simulink model "model_simscape"  (R2021a)
settings: Solver=VariableStepAuto  StartTime=0.0  StopTime=10  FixedStep=Ts  RelTol=1e-3
values from neighbouring files (symbols this model uses):
  acc_C = -1/g    (= -0.101936799185)    [params.m]
  acc_enable = 1    [params.m]
  acc_noise_var = 1e-10    [params.m]
  B_hs = 1e5    (= 100000)    [params.m]
  b_small_bot = 1400    [params.m]
  b_small_up = 1417.14082244839    (= 1417.14082245)    [params.m]
  beta = 0    [params.m]
  flow_C = flow_enable/flow_C_ratio/conv_SI    (= 59999.988)    [params.m]
  flow_C_ratio = dm_max/U_f_max    (= 1)    [params.m]
  flow_noise_var = 1e-10    [params.m]
  g = 9.81    [params.m]
  K_hs = 1e5    (= 100000)    [params.m]
  L = NaN(N,nk)    [hammerstein_wiener_model_estimation.m]    (also in params.m = 0.2)
  M = 6.7798462575453    (= 6.77984625755)    [params.m]
  M_L = member.("Settings.Load"){1,1}{1,1}    [identification_faultcode.m]    (also in params.m = 6.25)
  P_0 = 101325    [params.m]
  P_s = 6e5    (= 600000)    [params.m]
  prox_bot_band = 4e-4    (= 0.0004)    [params.m]
  prox_up_band = 0.1925    [params.m]
  SmallDamper_bottom = member.SmallDamper_bottom{1,1}.Variables    [identification_faultcode.m]    (also in params.m = 6)
  SmallDamper_upper = member.SmallDamper_upper{1,1}.Variables    [identification_faultcode.m]    (also in params.m = 4)
  T = cell2mat(T)    [data_driven_models_perfomance.m]    (also in params.m = 281.7)
  Ts = 1e-3    (= 0.001)    [data_driven_models_perfomance.m]    (also in hammerstein_wiener_model_estimation.m; params.m)
  valve1 = member.ThrottleValve2{1,1}.Variables    [identification_faultcode.m]    (also in params.m = 4)
  valve2 = member.ThrottleValve1{1,1}.Variables    [identification_faultcode.m]    (also in params.m = 6)
  x0 = 0    [params.m]
libraries: fl_lib x20, nesl_utility x14, SimscapeFluids_lib x6
(part 2 of 2)

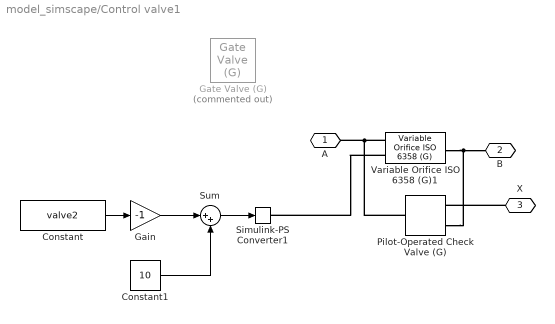
== system model_simscape/Control valve1 ==
  Constant : Constant  Value=valve2
  Constant1 : Constant  Value=10
  Gain : Gain  Gain=-1
  Gate Valve (G) : SimscapeFluids_lib/Gas/Valves & Orifices/Flow Control Valves/Gate Valve (G)  Commented=on  diam_orifice=d_G18 m  x0=0  iso_cond_spec=fluids.gas.enum.flow_control_valve_spec.Cv  C_max=1.6 l/s/bar  B_crit=0.3  m=0.5  Cv_max=0.53  Kv_max=0.3  area_leak=1e-12 m^2  area=cs_G18 m^2  smoothing_factor=0  B_lam=B_lam  T0=T K  rho0=rho kg/m^3
      settings: SourceProductBaseCode=SH  InternalSimscapePortConfiguration="{\"Bottom\":[],\"Left\":[{\"id\":\"A\",\"label\":\"A\",\"type\":\"foundation.gas.gas\"},{\"id\":\"L\",\"label\":\"L\",\"type\":\"input\"}],\"Right\":[{\"id\":\"B\",\"label\":\"B\",\"type\":\"foundation.gas.gas\"}],\"Top\":[]}"
  Pilot-Operated Check Valve (G) : SimscapeFluids_lib/Gas/Valves & Orifices/Directional Control Valves/Pilot-Operated Check Valve (G)  pressure_spec=fluids.gas.enum.pilot_pressure_control_spec.dp  p_crack_differential=6 bar  press_max_differential=7 bar  pilot_ratio=1  iso_cond_spec=fluids.gas.enum.iso_cond_spec.Kv  C_max=1.6 l/s/bar  C_min=1e-5 l/s/bar  B_crit=0.3  m=0.5  Cv_max=0.38  Cv_min=1e-6  Kv_max=0.3287  Kv_min=1e-6  area_max=1e-4 m^2  area_leak=1e-12 m^2  area=0.01 m^2  smoothing_factor=0  B_lam=0.999  T0=293.15 K  rho0=1.185 kg/m^3
      settings: SourceProductBaseCode=SH  InternalSimscapePortConfiguration="{\"Bottom\":[],\"Left\":[{\"id\":\"A\",\"label\":\"A\",\"type\":\"foundation.gas.gas\"},{\"id\":\"X\",\"label\":\"X\",\"type\":\"foundation.gas.gas\"}],\"Right\":[{\"id\":\"B\",\"label\":\"B\",\"type\":\"foundation.gas.gas\"}],\"Top\":[]}"
  Simulink-PS Converter1 : nesl_utility/Simulink-PS Converter  PhysicalDomain=network_engine_domain  SubClassName=ps_input  LeftPortType=input  RightPortType=output  PseudoPeriodic=off  Frequencies=[]  NoiseDistribution=none  NoiseParameters=[]  Unit=1  AffineConversion=off  FilteringAndDerivatives=provide  SimscapeFilterOrder=1  InputFilterTimeConstant=0.001  UdotUserProvided=0
      settings: SourceProductBaseCode=PW,SS
  Sum : Sum  Inputs=|++
  Variable Orifice ISO 6358 (G)1 : SimscapeFluids_lib/Gas/Valves & Orifices/Variable Orifice ISO 6358 (G)  iso_cond_spec=fluids.gas.enum.iso_cond_spec.Kv  iso_opening_spec_C=fluids.gas.enum.iso_opening_spec.linear  C_max=1.6 l/s/bar  C_min=1e-5 l/s/bar  B_crit=0.3  opening_C_TLU=0 : 0.2 : 1  C_TLU=[1e-05, .32, .64, .96, 1.28, 1.6] l/s/bar  B_crit_TLU=0.3 * ones(1, 6)  m=0.5  iso_opening_spec_Cv=fluids.gas.enum.iso_opening_spec.tabulated  Cv_max=0.4  Cv_min=1e-6  opening_Cv_TLU=0 : 0.2 : 1  Cv_TLU=[1e-06, .08, .16, .24, .32, .4]  iso_opening_spec_Kv=fluids.gas.enum.iso_opening_spec.tabulated  Kv_max=0.1038  Kv_min=Kv_min_cntr  opening_Kv_TLU=lookup_n  Kv_TLU=lookup_qn_Kv  iso_opening_spec_area=fluids.gas.enum.iso_opening_spec.linear  restriction_area_max=1e-5 m^2  restriction_area_min=1e-10 m^2  opening_area_TLU=0 : 0.2 : 1  restriction_area_TLU=[1e-10, 2e-06, 4e-06, 6e-06, 8e-06, 1e-05] m^2  area=cs_G18 m^2  B_lam=0.999  T0=T K  rho0=rho kg/m^3  smoothing_factor=0
      settings: SourceProductBaseCode=SH  InternalSimscapePortConfiguration="{\"Bottom\":[],\"Left\":[{\"id\":\"A\",\"label\":\"A\",\"type\":\"foundation.gas.gas\"},{\"id\":\"L\",\"label\":\"L\",\"type\":\"input\"}],\"Right\":[{\"id\":\"B\",\"label\":\"B\",\"type\":\"foundation.gas.gas\"}],\"Top\":[]}"
  A : PMIOPort  Side=Left
  B : PMIOPort  Port=2  Side=Right
  X : PMIOPort  Port=3  Side=Left
  wires:
  Sum/1 -> Simulink-PS Converter1/1
  Gain/1 -> Sum/1
  Constant/1 -> Gain/1
  Constant1/1 -> Sum/2
  connections:
  Variable Orifice ISO 6358 (G)1/LConn1 -- Pilot-Operated Check Valve (G)/RConn1 -- A/RConn1
  Variable Orifice ISO 6358 (G)1/RConn1 -- Pilot-Operated Check Valve (G)/LConn1 -- B/RConn1
  Variable Orifice ISO 6358 (G)1/LConn2 -- Simulink-PS Converter1/RConn1
  X/RConn1 -- Pilot-Operated Check Valve (G)/LConn2

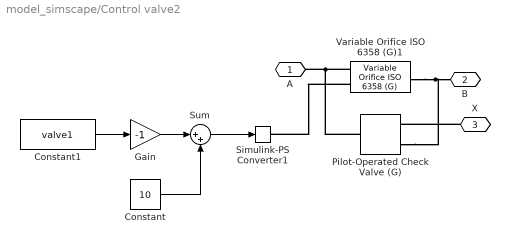
== system model_simscape/Control valve2 ==
  Constant : Constant  Value=10
  Constant1 : Constant  Value=valve1
  Gain : Gain  Gain=-1
  Pilot-Operated Check Valve (G) : SimscapeFluids_lib/Gas/Valves & Orifices/Directional Control Valves/Pilot-Operated Check Valve (G)  pressure_spec=fluids.gas.enum.pilot_pressure_control_spec.dp  p_crack_differential=6 bar  press_max_differential=7 bar  pilot_ratio=1  iso_cond_spec=fluids.gas.enum.iso_cond_spec.Kv  C_max=1.6 l/s/bar  C_min=1e-5 l/s/bar  B_crit=0.3  m=0.5  Cv_max=0.4  Cv_min=1e-6  Kv_max=0.3287  Kv_min=1e-6  area_max=1e-4 m^2  area_leak=1e-12 m^2  area=0.01 m^2  smoothing_factor=0  B_lam=0.999  T0=293.15 K  rho0=1.185 kg/m^3
      settings: SourceProductBaseCode=SH  InternalSimscapePortConfiguration="{\"Bottom\":[],\"Left\":[{\"id\":\"A\",\"label\":\"A\",\"type\":\"foundation.gas.gas\"},{\"id\":\"X\",\"label\":\"X\",\"type\":\"foundation.gas.gas\"}],\"Right\":[{\"id\":\"B\",\"label\":\"B\",\"type\":\"foundation.gas.gas\"}],\"Top\":[]}"
  Simulink-PS Converter1 : nesl_utility/Simulink-PS Converter  PhysicalDomain=network_engine_domain  SubClassName=ps_input  LeftPortType=input  RightPortType=output  PseudoPeriodic=off  Frequencies=[]  NoiseDistribution=none  NoiseParameters=[]  Unit=1  AffineConversion=off  FilteringAndDerivatives=provide  SimscapeFilterOrder=1  InputFilterTimeConstant=0.001  UdotUserProvided=0
      settings: SourceProductBaseCode=PW,SS
  Sum : Sum  Inputs=|++
  Variable Orifice ISO 6358 (G)1 : SimscapeFluids_lib/Gas/Valves & Orifices/Variable Orifice ISO 6358 (G)  iso_cond_spec=fluids.gas.enum.iso_cond_spec.Kv  iso_opening_spec_C=fluids.gas.enum.iso_opening_spec.linear  C_max=1.6 l/s/bar  C_min=1e-5 l/s/bar  B_crit=0.3  opening_C_TLU=0 : 0.2 : 1  C_TLU=[1e-05, .32, .64, .96, 1.28, 1.6] l/s/bar  B_crit_TLU=0.3 * ones(1, 6)  m=0.5  iso_opening_spec_Cv=fluids.gas.enum.iso_opening_spec.tabulated  Cv_max=0.4  Cv_min=1e-6  opening_Cv_TLU=0 : 0.2 : 1  Cv_TLU=[1e-06, .08, .16, .24, .32, .4]  iso_opening_spec_Kv=fluids.gas.enum.iso_opening_spec.tabulated  Kv_max=0.1038  Kv_min=Kv_min_cntr  opening_Kv_TLU=lookup_n  Kv_TLU=lookup_qn_Kv  iso_opening_spec_area=fluids.gas.enum.iso_opening_spec.linear  restriction_area_max=1e-5 m^2  restriction_area_min=1e-10 m^2  opening_area_TLU=0 : 0.2 : 1  restriction_area_TLU=[1e-10, 2e-06, 4e-06, 6e-06, 8e-06, 1e-05] m^2  area=cs_G18 m^2  B_lam=0.999  T0=T K  rho0=rho kg/m^3  smoothing_factor=0
      settings: SourceProductBaseCode=SH  InternalSimscapePortConfiguration="{\"Bottom\":[],\"Left\":[{\"id\":\"A\",\"label\":\"A\",\"type\":\"foundation.gas.gas\"},{\"id\":\"L\",\"label\":\"L\",\"type\":\"input\"}],\"Right\":[{\"id\":\"B\",\"label\":\"B\",\"type\":\"foundation.gas.gas\"}],\"Top\":[]}"
  A : PMIOPort  Side=Left
  B : PMIOPort  Port=2  Side=Right
  X : PMIOPort  Port=3  Side=Left
  wires:
  Constant1/1 -> Gain/1
  Sum/1 -> Simulink-PS Converter1/1
  Constant/1 -> Sum/2
  Gain/1 -> Sum/1
  connections:
  Variable Orifice ISO 6358 (G)1/LConn1 -- Pilot-Operated Check Valve (G)/RConn1 -- A/RConn1
  Variable Orifice ISO 6358 (G)1/RConn1 -- Pilot-Operated Check Valve (G)/LConn1 -- B/RConn1
  X/RConn1 -- Pilot-Operated Check Valve (G)/LConn2
  Variable Orifice ISO 6358 (G)1/LConn2 -- Simulink-PS Converter1/RConn1

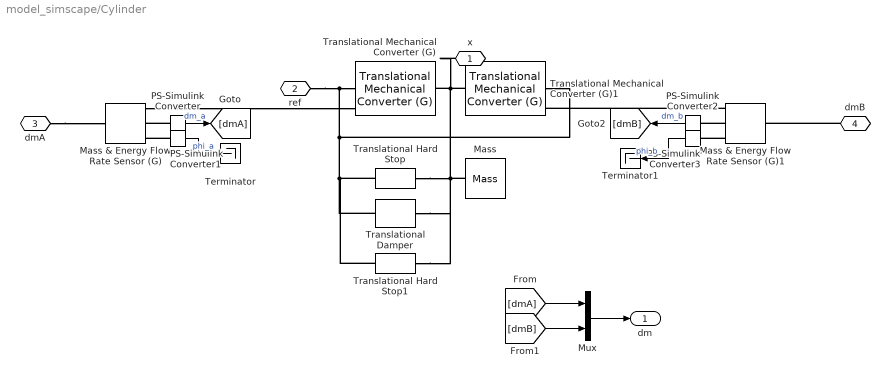
== system model_simscape/Cylinder ==
  Mass : fl_lib/Mechanical/Translational Elements/Mass  mass=M+M_L kg  num_ports=foundation.enum.numPorts2.one  v_specify=off  v_priority=High  v=0 m/s  v_nominal_specify=off  v_nominal_unit=m/s  v_nominal_value=1  f_specify=off  f_priority=None  f=0 N  f_nominal_specify=off  f_nominal_unit=N  f_nominal_value=1
  Mass & Energy Flow Rate Sensor (G) : fl_lib/Gas/Sensors/Mass & Energy Flow Rate Sensor (G)
      settings: SourceProductBaseCode=SS  InternalSimscapePortConfiguration="{\"Bottom\":[],\"Left\":[{\"id\":\"A\",\"label\":\"A\",\"type\":\"foundation.gas.gas\"}],\"Right\":[{\"id\":\"B\",\"label\":\"B\",\"type\":\"foundation.gas.gas\"},{\"id\":\"M\",\"label\":\"M\",\"type\":\"output\"},{\"id\":\"PHI\",\"label\":\"Phi\",\"type\":\"output\"}],\"Top\":[]}"
  Mass & Energy Flow Rate Sensor (G)1 : fl_lib/Gas/Sensors/Mass & Energy Flow Rate Sensor (G)
      settings: SourceProductBaseCode=SS  InternalSimscapePortConfiguration="{\"Bottom\":[],\"Left\":[{\"id\":\"A\",\"label\":\"A\",\"type\":\"foundation.gas.gas\"}],\"Right\":[{\"id\":\"B\",\"label\":\"B\",\"type\":\"foundation.gas.gas\"},{\"id\":\"M\",\"label\":\"M\",\"type\":\"output\"},{\"id\":\"PHI\",\"label\":\"Phi\",\"type\":\"output\"}],\"Top\":[]}"
  Mux : Mux  Inputs=2
  PS-Simulink Converter{,1..3} (4 alike) : nesl_utility/PS-Simulink Converter  PhysicalDomain=network_engine_domain  SubClassName=ps_output  LeftPortType=input  RightPortType=output  PseudoPeriodic=off  Frequencies=[]  Unit=inherit  AffineConversion=off
      settings: SourceProductBaseCode=PW,SS
  Terminator : Terminator
  Terminator1 : Terminator
  Translational Mechanical Converter (G) : fl_lib/Gas/Elements/Translational Mechanical Converter (G)  mech_orientation=simscape.enum.posneg.positive  displacement_spec=foundation.enum.DisplacementSpec.Calculate  length_init=x0 m  interface_area=S_A m^2  dead_volume=V_0A m^3  area_A=cs_A m^2  environment_spec=foundation.enum.pressure_spec.atmospheric  environment_pressure=0.101325 MPa  p_I_specify=on  p_I_priority=High  p_I=0.101325 MPa  p_I_nominal_specify=off  p_I_nominal_unit=MPa  p_I_nominal_value=1  T_I_specify=on  T_I_priority=High  T_I=293.15 K  T_I_nominal_specify=off  T_I_nominal_unit=K  T_I_nominal_value=1  rho_converter_specify=off  rho_converter_priority=None  rho_converter=1.2 kg/m^3  rho_converter_nominal_specify=off  rho_converter_nominal_unit=kg/m^3  rho_converter_nominal_value=1
      settings: SourceProductBaseCode=SS  InternalSimscapePortConfiguration="{\"Bottom\":[],\"Left\":[{\"id\":\"A\",\"label\":\"A\",\"type\":\"foundation.gas.gas\"},{\"id\":\"C\",\"label\":\"C\",\"type\":\"foundation.mechanical.translational.translational\"},{\"id\":\"H\",\"label\":\"H\",\"type\":\"foundation.thermal.thermal\"}],\"Right\":[{\"id\":\"R\",\"label\":\"R\",\"type\":\"foundation.mechanical.translational.translational\"}],\"Top\":[]}"
  Translational Mechanical Converter (G)1 : fl_lib/Gas/Elements/Translational Mechanical Converter (G)  mech_orientation=simscape.enum.posneg.negative  displacement_spec=foundation.enum.DisplacementSpec.Calculate  length_init=-L+x0 m  interface_area=S_B m^2  dead_volume=V_0B m^3  area_A=cs_B m^2  environment_spec=foundation.enum.pressure_spec.atmospheric  environment_pressure=0.101325 MPa  p_I_specify=on  p_I_priority=High  p_I=0.101325 MPa  p_I_nominal_specify=off  p_I_nominal_unit=MPa  p_I_nominal_value=1  T_I_specify=on  T_I_priority=High  T_I=293.15 K  T_I_nominal_specify=off  T_I_nominal_unit=K  T_I_nominal_value=1  rho_converter_specify=off  rho_converter_priority=None  rho_converter=1.2 kg/m^3  rho_converter_nominal_specify=off  rho_converter_nominal_unit=kg/m^3  rho_converter_nominal_value=1
      settings: SourceProductBaseCode=SS  InternalSimscapePortConfiguration="{\"Bottom\":[],\"Left\":[{\"id\":\"A\",\"label\":\"A\",\"type\":\"foundation.gas.gas\"},{\"id\":\"C\",\"label\":\"C\",\"type\":\"foundation.mechanical.translational.translational\"},{\"id\":\"H\",\"label\":\"H\",\"type\":\"foundation.thermal.thermal\"}],\"Right\":[{\"id\":\"R\",\"label\":\"R\",\"type\":\"foundation.mechanical.translational.translational\"}],\"Top\":[]}"
  Translational Damper : fl_lib/Mechanical/Translational Elements/Translational Damper  D=beta N/(m/s)  v_specify=off  v_priority=None  v=0 m/s  v_nominal_specify=off  v_nominal_unit=m/s  v_nominal_value=1  f_specify=off  f_priority=None  f=0 N  f_nominal_specify=off  f_nominal_unit=N  f_nominal_value=1
  Translational Hard Stop : fl_lib/Mechanical/Translational Elements/Translational Hard Stop  upper_bnd=gp m  lower_bnd=gn m  stiff_up=K_hs*1e3 N/m  stiff_low=K_hs*1e3 N/m  D_up=B_hs*1e3 N/(m/s)  D_low=B_hs*1e3 N/(m/s)  model=simscape.enum.hardstop.fullundamped  transition=tr_hs mm  v_specify=off  v_priority=None  v=0 m/s  v_nominal_specify=off  v_nominal_unit=m/s  v_nominal_value=1  f_specify=off  f_priority=None  f=0 N  f_nominal_specify=off  f_nominal_unit=N  f_nominal_value=1  x_specify=on  x_priority=High  x=x0 m  x_nominal_specify=off  x_nominal_unit=m  x_nominal_value=1
  Translational Hard Stop1 : fl_lib/Mechanical/Translational Elements/Translational Hard Stop  upper_bnd=up_damp_start m  lower_bnd=bot_damp_start m  stiff_up=0 N/m  stiff_low=0 N/m  D_up=b_small_up * SmallDamper_upper N/(m/s)  D_low=b_small_bot * SmallDamper_bottom N/(m/s)  model=simscape.enum.hardstop.fullundamped  transition=tr_reg mm  v_specify=on  v_priority=None  v=0 m/s  v_nominal_specify=off  v_nominal_unit=m/s  v_nominal_value=1  f_specify=off  f_priority=None  f=0 N  f_nominal_specify=off  f_nominal_unit=N  f_nominal_value=1  x_specify=on  x_priority=High  x=x0 m  x_nominal_specify=off  x_nominal_unit=m  x_nominal_value=1
  x : PMIOPort  Side=Right
  ref : PMIOPort  Port=2  Side=Left
  dmA : PMIOPort  Port=3  Side=Left
  dmB : PMIOPort  Port=4  Side=Left
  dm : Outport
  wires:
  PS-Simulink Converter/1 -> [dmA]  "dm_a"
  PS-Simulink Converter2/1 -> [dmB]  "dm_b"
  PS-Simulink Converter1/1 -> Terminator/1  "phi_a"
  PS-Simulink Converter3/1 -> Terminator1/1  "phi_b"
  [dmB] -> Mux/2
  [dmA] -> Mux/1
  Mux/1 -> dm/1
  connections:
  Translational Mechanical Converter (G)1/RConn1 -- x/RConn1 -- Translational Hard Stop1/LConn1 -- Translational Damper/LConn1 -- Translational Hard Stop/LConn1 -- Mass/LConn1 -- Translational Mechanical Converter (G)/RConn1
  Translational Mechanical Converter (G)1/LConn2 -- Translational Hard Stop1/RConn1 -- Translational Damper/RConn1 -- Translational Hard Stop/RConn1 -- ref/RConn1 -- Translational Mechanical Converter (G)/LConn2
  PS-Simulink Converter/LConn1 -- Mass & Energy Flow Rate Sensor (G)/RConn2
  PS-Simulink Converter1/LConn1 -- Mass & Energy Flow Rate Sensor (G)/RConn3
  Mass & Energy Flow Rate Sensor (G)1/RConn3 -- PS-Simulink Converter3/LConn1
  Mass & Energy Flow Rate Sensor (G)1/RConn2 -- PS-Simulink Converter2/LConn1
  Mass & Energy Flow Rate Sensor (G)/RConn1 -- Translational Mechanical Converter (G)/LConn1
  dmA/RConn1 -- Mass & Energy Flow Rate Sensor (G)/LConn1
  Mass & Energy Flow Rate Sensor (G)1/RConn1 -- Translational Mechanical Converter (G)1/LConn1
  dmB/RConn1 -- Mass & Energy Flow Rate Sensor (G)1/LConn1

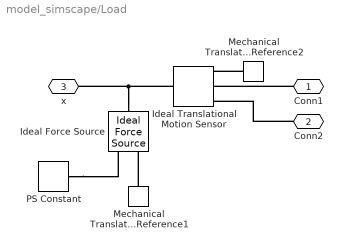
== system model_simscape/Load ==
  Ideal Force Source : fl_lib/Mechanical/Mechanical Sources/Ideal Force Source
  Ideal Translational Motion Sensor : fl_lib/Mechanical/Mechanical Sensors/Ideal Translational Motion Sensor  offset=x0 m
  Mechanical Translational Reference1 : fl_lib/Mechanical/Translational Elements/Mechanical Translational Reference
  Mechanical Translational Reference2 : fl_lib/Mechanical/Translational Elements/Mechanical Translational Reference
  PS Constant : fl_lib/Physical Signals/Sources/PS Constant  constant=-(M+M_L)*g N
  Conn1 : PMIOPort  Side=Right
  Conn2 : PMIOPort  Port=2  Side=Right
  x : PMIOPort  Port=3  Side=Left
  connections:
  Conn2/RConn1 -- Ideal Translational Motion Sensor/RConn3
  Conn1/RConn1 -- Ideal Translational Motion Sensor/RConn2
  Mechanical Translational Reference1/LConn1 -- Ideal Force Source/RConn2
  Ideal Translational Motion Sensor/LConn1 -- x/RConn1 -- Ideal Force Source/LConn1
  Mechanical Translational Reference2/LConn1 -- Ideal Translational Motion Sensor/RConn1
  PS Constant/RConn1 -- Ideal Force Source/RConn1

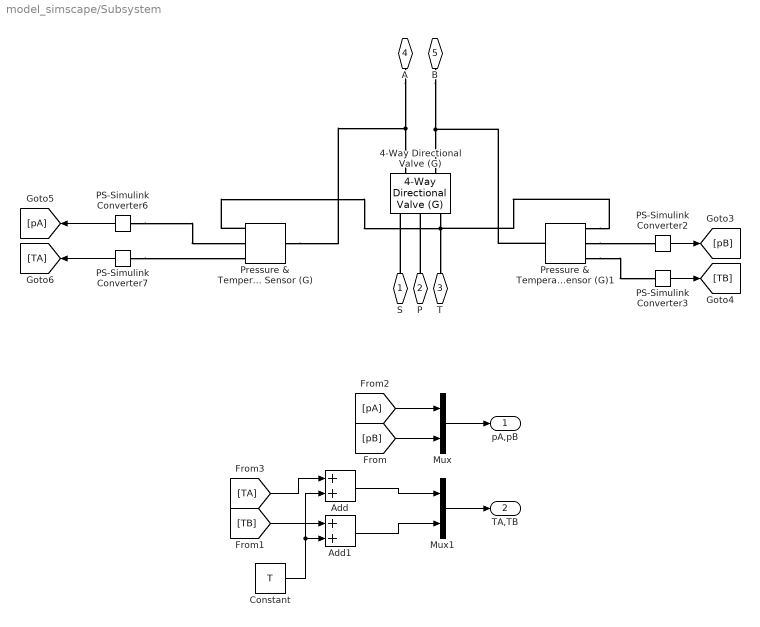
== system model_simscape/Subsystem ==
  4-Way Directional Valve (G) : SimscapeFluids_lib/Gas/Valves & Orifices/Directional Control Valves/4-Way Directional Valve (G)  iso_cond_spec=fluids.gas.enum.iso_cond_spec.Kv  iso_opening_spec_C=fluids.gas.enum.iso_opening_spec.linear  C_max=1.6 l/s/bar  C_min=1e-5 l/s/bar  B_crit=0.3  opening_C_TLU=0 : 0.2 : 1  C_TLU=[1e-05, .32, .64, .96, 1.28, 1.6] l/s/bar  B_crit_TLU=0.3 * ones(1, 6)  m=0.5  iso_opening_spec_Cv=fluids.gas.enum.iso_opening_spec.linear  Cv_max=1.03  Cv_min=1e-6  opening_Cv_TLU=0 : 0.2 : 1  Cv_TLU=[1e-06, .08, .16, .24, .32, .4]  iso_opening_spec_Kv=fluids.gas.enum.iso_opening_spec.linear  Kv_max=Kv_max_main  Kv_min=Kv_min_main  opening_Kv_TLU=0 : 0.2 : 1  Kv_TLU=[1e-06, .06, .12, .18, .24, .3]  iso_opening_spec_area=fluids.gas.enum.iso_opening_spec.linear  restriction_area_max=1e-5 m^2  restriction_area_min=1e-10 m^2  opening_area_TLU=0 : 0.2 : 1  restriction_area_TLU=[1e-10, 2e-06, 4e-06, 6e-06, 8e-06, 1e-05] m^2  area=cs_G18 m^2  smoothing_factor=0  B_lam=B_lam  T0=T K  rho0=rho kg/m^3  x0_P_A=H_P2A  x0_B_T=H_B2T  x0_P_B=H_P2B  x0_A_T=H_A2T
      settings: SourceProductBaseCode=SH  InternalSimscapePortConfiguration="{\"Bottom\":[],\"Left\":[{\"id\":\"A\",\"label\":\"A\",\"type\":\"foundation.gas.gas\"},{\"id\":\"B\",\"label\":\"B\",\"type\":\"foundation.gas.gas\"}],\"Right\":[{\"id\":\"S\",\"label\":\"S\",\"type\":\"input\"},{\"id\":\"P\",\"label\":\"P\",\"type\":\"foundation.gas.gas\"},{\"id\":\"T\",\"label\":\"T\",\"type\":\"foundation.gas.gas\"}],\"Top\":[]}"
  Add : Sum
  Add1 : Sum
  Constant : Constant  Value=T
  Mux : Mux  Inputs=2
  Mux1 : Mux  Inputs=2
  PS-Simulink Converter{2..3,6..7} (4 alike) : nesl_utility/PS-Simulink Converter  PhysicalDomain=network_engine_domain  SubClassName=ps_output  LeftPortType=input  RightPortType=output  PseudoPeriodic=off  Frequencies=[]  Unit=inherit  AffineConversion=off
      settings: SourceProductBaseCode=PW,SS
  Pressure & Temperature Sensor (G) : fl_lib/Gas/Sensors/Pressure & Temperature Sensor (G)
      settings: SourceProductBaseCode=SS  InternalSimscapePortConfiguration="{\"Bottom\":[],\"Left\":[{\"id\":\"A\",\"label\":\"A\",\"type\":\"foundation.gas.gas\"}],\"Right\":[{\"id\":\"B\",\"label\":\"B\",\"type\":\"foundation.gas.gas\"},{\"id\":\"P\",\"label\":\"P\",\"type\":\"output\"},{\"id\":\"T\",\"label\":\"T\",\"type\":\"output\"}],\"Top\":[]}"
  Pressure & Temperature Sensor (G)1 : fl_lib/Gas/Sensors/Pressure & Temperature Sensor (G)
      settings: SourceProductBaseCode=SS  InternalSimscapePortConfiguration="{\"Bottom\":[],\"Left\":[{\"id\":\"A\",\"label\":\"A\",\"type\":\"foundation.gas.gas\"}],\"Right\":[{\"id\":\"B\",\"label\":\"B\",\"type\":\"foundation.gas.gas\"},{\"id\":\"P\",\"label\":\"P\",\"type\":\"output\"},{\"id\":\"T\",\"label\":\"T\",\"type\":\"output\"}],\"Top\":[]}"
  S : PMIOPort  Side=Right
  P : PMIOPort  Port=2  Side=Right
  T : PMIOPort  Port=3  Side=Right
  A : PMIOPort  Port=4  Side=Left
  B : PMIOPort  Port=5  Side=Left
  pA,pB : Outport
  TA,TB : Outport  Port=2
  wires:
  PS-Simulink Converter3/1 -> [TB]
  PS-Simulink Converter6/1 -> [pA]
  PS-Simulink Converter7/1 -> [TA]
  PS-Simulink Converter2/1 -> [pB]
  [pA] -> Mux/1
  [pB] -> Mux/2
  Mux/1 -> pA,pB/1
  Mux1/1 -> TA,TB/1
  [TA] -> Add/1
  Add/1 -> Mux1/1
  Add1/1 -> Mux1/2
  [TB] -> Add1/1
  Constant/1 -> Add/2, Add1/2
  connections:
  Pressure & Temperature Sensor (G)1/RConn3 -- PS-Simulink Converter3/LConn1
  S/RConn1 -- 4-Way Directional Valve (G)/RConn1
  B/RConn1 -- Pressure & Temperature Sensor (G)1/LConn1 -- 4-Way Directional Valve (G)/LConn2
  PS-Simulink Converter7/LConn1 -- Pressure & Temperature Sensor (G)/RConn3
  P/RConn1 -- 4-Way Directional Valve (G)/RConn2
  A/RConn1 -- Pressure & Temperature Sensor (G)/LConn1 -- 4-Way Directional Valve (G)/LConn1
  PS-Simulink Converter6/LConn1 -- Pressure & Temperature Sensor (G)/RConn2
  Pressure & Temperature Sensor (G)1/RConn2 -- PS-Simulink Converter2/LConn1
  4-Way Directional Valve (G)/RConn3 -- T/RConn1 -- Pressure & Temperature Sensor (G)/RConn1 -- Pressure & Temperature Sensor (G)1/RConn1

== matlab function model_simscape/AccelerometerMoving_axisZ ==
  settings: updateMethod=DISCRETE  sampleTime=Ts
  data: ddx input; acc output; acc_noise_var parameter; acc_enable parameter; acc_C parameter
function acc = fcn(ddx, acc_noise_var, acc_enable, acc_C)

acc = acc_enable * acc_C * ddx + acc_noise_var * rand() + 1;
end

== matlab function model_simscape/MATLAB Function ==
  data: dm input; dm_in output; dm_out output
function [dm_in, dm_out]= fcn(dm)
if dm > 0
    dm_in = dm;
    dm_out = 0;
elseif dm < 0
    dm_in = 0;
    dm_out = abs(dm);
else
    dm_in = 0;
    dm_out = 0;
end
end

== matlab function model_simscape/Flow_sensor ==
  settings: updateMethod=DISCRETE
  data: dm_A input; dm_A_sensor output; flow_C parameter; flow_C_ratio parameter; flow_noise_var parameter
function dm_A_sensor = fcn(dm_A, flow_C, flow_C_ratio, flow_noise_var)
dm_A_sensor = flow_C*(flow_C_ratio*dm_A + flow_noise_var*rand());

== matlab function model_simscape/Proximity sensor ==
  data: x input; up output; bot output; prox_up_band parameter; prox_bot_band parameter
function [up,bot]= fcn(x, prox_up_band, prox_bot_band)
if x >= prox_up_band
    up = 1; bot = 0;
elseif x <= prox_bot_band
    bot = 1; up = 0;
else
    bot = 0;
    up = 0;
end

== matlab function model_simscape/Flow_sensor1 ==
  settings: updateMethod=DISCRETE
  data: dm_A input; dm_A_sensor output; flow_C parameter; flow_C_ratio parameter; flow_noise_var parameter
function dm_A_sensor = fcn(dm_A, flow_C, flow_C_ratio, flow_noise_var)
dm_A_sensor = flow_C*(flow_C_ratio*dm_A + flow_noise_var*rand());
